simulink model "Logistic"  (Simulink 6.6)
settings: Solver=ode45  StartTime=0.0  StopTime=10.0  RelTol=1e-3
settings Model: Creator=mxkana  LastModifiedBy=mxkana

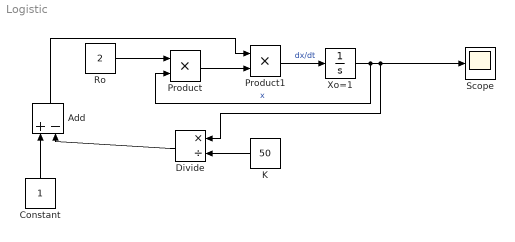
== system Logistic ==
  Add : Sum  Orientation=up  Inputs=+-  OutScaling=2^-10
  Constant : Constant  Orientation=up
  Divide : Product  Orientation=left  Inputs=*/  OutScaling=2^-10
  K : Constant  Orientation=left  Value=50
  Product : Product  RndMeth=Zero
  Product1 : Product  RndMeth=Zero
  Ro : Constant  Value=2
  Scope : Scope
      settings: YMin=0  YMax=100
  Xo=1 : Integrator  InitialCondition=1
  wires:
  Constant/1 -> Add/1
  Ro/1 -> Product/1
  Product1/1 -> Xo=1/1  "dx/dt"
  Product/1 -> Product1/2
  Xo=1/1 -> Divide/1, Scope/1, Product/2  "x"
  K/1 -> Divide/2
  Divide/1 -> Add/2
  Add/1 -> Product1/1
